simulink model "simF16_u02"  (R2023b)
settings: Solver=ode4  StartTime=0  StopTime=15  FixedStep=0.005  RelTol=1e-3  EnableMultiTasking=on
values from neighbouring files (symbols this model uses):
  control_trim = u0    [find_trim.m]    (also in trimcond.mat = [0.154059600013 -0.694715670316 -3.42749873112e-15 4.5481145; trimcond2.mat = [0.154007747083 -0.694801754663 0.00182544197392 0.000329744)
  state_trim = constraint( state )    [find_trim.m]    (also in trimcond.mat = [502 0.0505701217863 2.65111802467e-16 0 0.0505701217863 0 0; trimcond2.mat = [501.999976668 0.0505473192089 -2.30406790676e-05 0.00010278)
settings Model: Creator=keviczky  LastModifiedBy=suvo
settings DataIOCC: Decimation=50  SaveFormat=Array  SignalLoggingSaveFormat=ModelDataLogs  ReturnWorkspaceOutputs=off  SignalLoggingName=sigsOut
settings OptimizationCC: BooleanDataType=off
settings DebuggingCC: SaveWithParameterizedLinksMsg=none  UnderspecifiedInitializationDetection=Classic  MergeDetectMultiDrivingBlocksExec=none  SignalResolutionControl=TryResolveAllWithWarning  MultiTaskDSMMsg=warning  MultiTaskCondExecSysMsg=none  UnconnectedInputMsg=warning  UnconnectedOutputMsg=warning  UnconnectedLineMsg=warning
settings HardwareCC: ProdBitPerPointer=32  ProdBitPerSizeT=32  ProdBitPerPtrDiffT=32  ProdLargestAtomicFloat=None  ProdIntDivRoundTo=Undefined  ProdEndianess=Unspecified  ProdWordSize=32  ProdHWDeviceType=32-bit Generic  TargetUnknown=on
settings ModelReferenceCC: PropagateSignalLabelsOutOfModel=off
settings GRTTargetCC: CombineOutputUpdateFcns=off  GRTInterface=on
settings ConfigComp: CovMetricSettings=dw  CovSaveCumulativeToWorkspaceVar=on  CovSaveSingleToWorkspaceVar=on

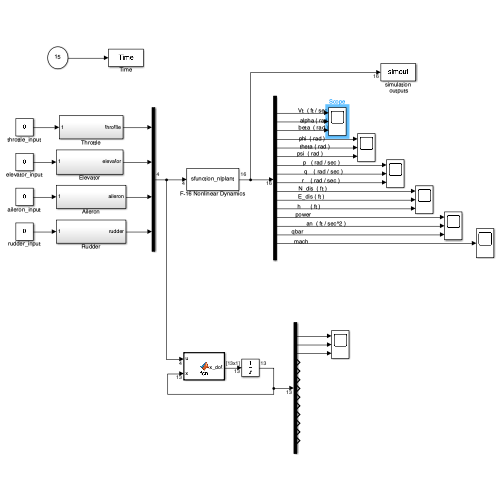
[thumbnail: Simulink's stored preview of the top-level diagram]
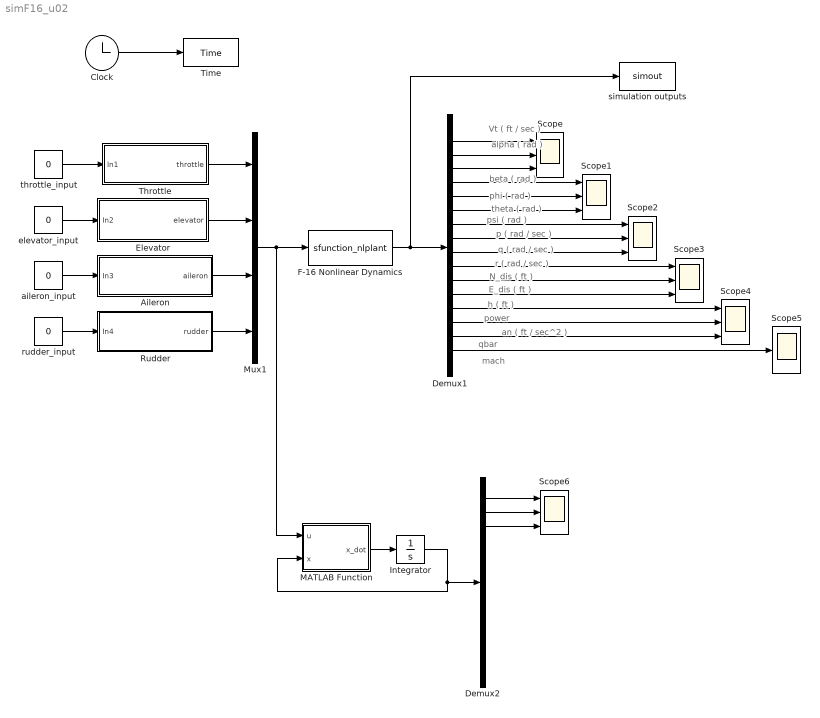
== system simF16_u02 ==
  note: Vt ( ft / sec )
  note: alpha ( rad )
  note: beta ( rad )
  note: phi ( rad )
  note: theta ( rad )
  note: psi ( rad )
  note: p ( rad / sec )
  note: q ( rad / sec )
  note: r ( rad / sec )
  note: N_dis ( ft )
  note: E_dis ( ft )
  note: h ( ft )
  note: power
  note: an ( ft / sec^2 )
  note: qbar
  note: mach
  Aileron : Subsystem
  Clock : Clock
      settings: Decimation=50
  Demux1 : Demux  Outputs=16
  Demux2 : Demux  Outputs=13
  Elevator : Subsystem
  F-16 Nonlinear Dynamics : S-Function  FunctionName=sfunction_nlplant  Parameters="state_trim,  xcg"  SFunctionDeploymentMode=off  EnableBusSupport=off
  Integrator : Integrator  InitialCondition=[state_trim]
  MATLAB Function : MATLAB Function  TreatAsAtomicUnit=on
  Mux1 : Mux
  Rudder : Subsystem
  Scope{,1..4,6} (6 alike) : Scope  NumInputPorts=3
  Scope5 : Scope
  Throttle : Subsystem
  Time : ToWorkspace  VariableName=Time  SampleTime=-1
      settings: Decimation=100
  aileron_input : Constant  Value=0
  elevator_input : Constant  Value=0
  rudder_input : Constant  Value=0
  simulation outputs : ToWorkspace  VariableName=simout  SampleTime=-1
      settings: Decimation=100
  throttle_input : Constant  Value=0
  wires:
  F-16 Nonlinear Dynamics/1 -> Demux1/1, simulation outputs/1
  Clock/1 -> Time/1
  Demux1/1 -> Scope/1
  Demux1/2 -> Scope/2
  Demux1/3 -> Scope/3
  Demux1/5 -> Scope1/2
  Demux1/6 -> Scope1/3
  Demux1/7 -> Scope2/1
  Demux1/8 -> Scope2/2
  Demux1/9 -> Scope2/3
  Demux1/10 -> Scope3/1
  Demux1/11 -> Scope3/2
  Demux1/12 -> Scope3/3
  Demux1/13 -> Scope4/1
  Demux1/14 -> Scope4/2
  Demux1/4 -> Scope1/1
  Demux1/15 -> Scope4/3
  Demux1/16 -> Scope5/1
  Throttle/1(throttle) -> Mux1/1
  Elevator/1(elevator) -> Mux1/2
  Aileron/1(aileron) -> Mux1/3
  Rudder/1(rudder) -> Mux1/4
  throttle_input/1 -> Throttle/1(In1)
  elevator_input/1 -> Elevator/1(In2)
  aileron_input/1 -> Aileron/1(In3)
  rudder_input/1 -> Rudder/1(In4)
  MATLAB Function/1(x_dot) -> Integrator/1
  Integrator/1 -> MATLAB Function/2(x), Demux2/1
  Mux1/1 -> MATLAB Function/1(u), F-16 Nonlinear Dynamics/1
  Demux2/1 -> Scope6/1
  Demux2/2 -> Scope6/2
  Demux2/3 -> Scope6/3

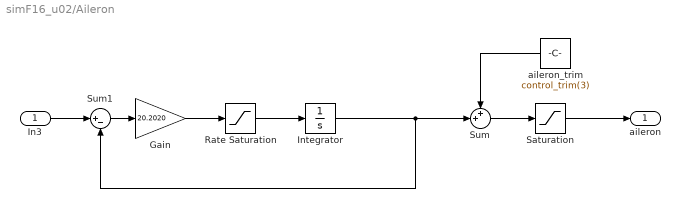
== system simF16_u02/Aileron ==
  In3 : Inport
  Gain : Gain  Gain=20.2020  SaturateOnIntegerOverflow=on  OutDataTypeStr=Inherit: Same as input  ParamDataTypeStr=Inherit: Same as input
  Integrator : Integrator  UpperSaturationLimit=21.5  LowerSaturationLimit=-21.5
  Rate Saturation : Saturate  UpperLimit=80  LowerLimit=-80
  Saturation : Saturate  UpperLimit=21.5  LowerLimit=-21.5
  Sum : Sum  Inputs=++|  InputSameDT=on  SaturateOnIntegerOverflow=on  OutDataTypeStr=Inherit: Same as first input
  Sum1 : Sum  Inputs=|+-  InputSameDT=on  SaturateOnIntegerOverflow=on  OutDataTypeStr=Inherit: Same as first input
  aileron_trim : Constant  Value=control_trim(3)
  aileron : Outport
  wires:
  In3/1 -> Sum1/1
  Sum1/1 -> Gain/1
  Gain/1 -> Rate Saturation/1
  Rate Saturation/1 -> Integrator/1
  Integrator/1 -> Sum1/2, Sum/2
  Sum/1 -> Saturation/1
  aileron_trim/1 -> Sum/1
  Saturation/1 -> aileron/1

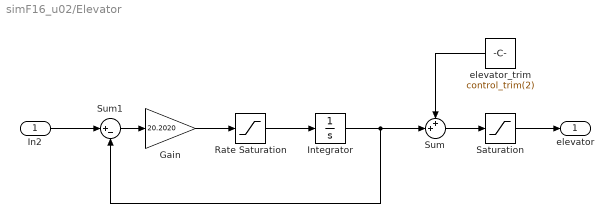
== system simF16_u02/Elevator ==
  In2 : Inport
  Gain : Gain  Gain=20.2020  SaturateOnIntegerOverflow=on  OutDataTypeStr=Inherit: Same as input  ParamDataTypeStr=Inherit: Same as input
  Integrator : Integrator  UpperSaturationLimit=25  LowerSaturationLimit=-25
  Rate Saturation : Saturate  UpperLimit=60  LowerLimit=-60
  Saturation : Saturate  UpperLimit=25  LowerLimit=-25
  Sum : Sum  Inputs=++|  InputSameDT=on  SaturateOnIntegerOverflow=on  OutDataTypeStr=Inherit: Same as first input
  Sum1 : Sum  Inputs=|+-  InputSameDT=on  SaturateOnIntegerOverflow=on  OutDataTypeStr=Inherit: Same as first input
  elevator_trim : Constant  Value=control_trim(2)
  elevator : Outport
  wires:
  In2/1 -> Sum1/1
  Sum1/1 -> Gain/1
  Gain/1 -> Rate Saturation/1
  Rate Saturation/1 -> Integrator/1
  Integrator/1 -> Sum1/2, Sum/2
  Sum/1 -> Saturation/1
  elevator_trim/1 -> Sum/1
  Saturation/1 -> elevator/1

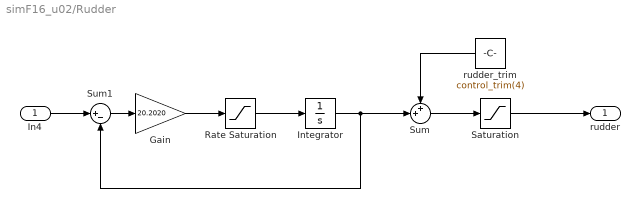
== system simF16_u02/Rudder ==
  In4 : Inport
  Gain : Gain  Gain=20.2020  SaturateOnIntegerOverflow=on  OutDataTypeStr=Inherit: Same as input  ParamDataTypeStr=Inherit: Same as input
  Integrator : Integrator  UpperSaturationLimit=30  LowerSaturationLimit=-30
  Rate Saturation : Saturate  UpperLimit=120  LowerLimit=-120
  Saturation : Saturate  UpperLimit=30  LowerLimit=-30
  Sum : Sum  Inputs=++|  InputSameDT=on  SaturateOnIntegerOverflow=on  OutDataTypeStr=Inherit: Same as first input
  Sum1 : Sum  Inputs=|+-  InputSameDT=on  SaturateOnIntegerOverflow=on  OutDataTypeStr=Inherit: Same as first input
  rudder_trim : Constant  Value=control_trim(4)
  rudder : Outport
  wires:
  In4/1 -> Sum1/1
  Sum1/1 -> Gain/1
  Gain/1 -> Rate Saturation/1
  Rate Saturation/1 -> Integrator/1
  Integrator/1 -> Sum1/2, Sum/2
  Saturation/1 -> rudder/1
  Sum/1 -> Saturation/1
  rudder_trim/1 -> Sum/1

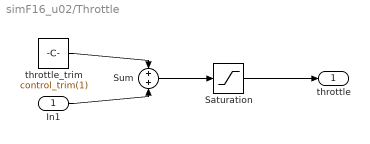
== system simF16_u02/Throttle ==
  In1 : Inport
  Saturation : Saturate  UpperLimit=1  LowerLimit=0
  Sum : Sum  InputSameDT=on  SaturateOnIntegerOverflow=on  OutDataTypeStr=Inherit: Same as first input
  throttle_trim : Constant  Value=control_trim(1)
  throttle : Outport
  wires:
  throttle_trim/1 -> Sum/1
  In1/1 -> Sum/2
  Sum/1 -> Saturation/1
  Saturation/1 -> throttle/1

== matlab function simF16_u02/MATLAB Function ==
  data: u input; x input; x_dot output
function x_dot = fcn(u,x)
%% ---- constant variable ----------------
s = 300;
b = 30;
cbar = 11.32;
rm = 1.57e-3; % 1 / mass
xcgr = 0.35;
he = 160.0;

x_dot = zeros(13,1);
xcg = 0.35;
control = u;

%% ---- Inertia constants ----------------
c1 = -0.770;
c2 = 0.02755;
c3 = 1.055e-4;
c4 = 1.642e-6;
c5 = 0.9604;
c6 = 1.759e-2;
c7 = 1.792e-5;
c8 = -0.7336;
c9 = 1.587e-5;

rtod = 180 / pi; %% radians to degrees
g = 32.174;

%% ---- Assign state variables ---------------
vt = x(1);
alpha = x(2) * rtod; %% x(2) in radians, alpha in degrees.
beta = x(3) * rtod;  %% x(3) in radians, beta in degrees.
phi = x(4);
theta = x(5);
psi = x(6);
p = x(7);
q = x(8);
r = x(9);
alt = x(12);
pow = x(13); % power

%% ---- Assign state & control variables ---------------
thtl = control(1);
el   = control(2);
ail  = control(3);
rdr  = control(4);

%% ---- Air Data computer and engine model ------------
[tfac, t, rho, amach, qbar, ps ] = adc ( vt, alt ); 
cpow = tgear (thtl);
x_dot (13) = pdot ( pow, cpow );  %% x_dot(13) = power derivative
t = thrust ( pow, alt, amach );

%% ---- Look-up tables and component biuldup ------------
cxt = cx ( alpha, el );
cyt = cy ( beta, ail, rdr );
czt = cz ( alpha, beta, el );
dail = ail / 20.0;
drdr = rdr / 30.0;
dlda_value = dlda( alpha, beta );
dldr_value = dldr( alpha, beta );
clt = cl( alpha, beta ) + dlda_value * dail + dldr_value * drdr;
cmt = cm( alpha, el );
dnda_value = dnda( alpha, beta );
dndr_value = dndr( alpha, beta );
cnt = cn( alpha, beta ) + dnda_value * dail + dndr_value * drdr;

%% ---- Add damping derivatives ------------
tvt = 0.5 / vt;
b2v = b * tvt;
cq = cbar * q * tvt;
d = damping( alpha );
cxt = cxt + cq * d(1);
cyt = cyt + b2v * ( d(2) * r + d(3) * p );
czt = czt + cq * d(4);
clt = clt + b2v * ( d(5) * r + d(6) * p );
cmt = cmt + cq * d(7) + czt * ( xcgr - xcg );
cnt = cnt + b2v * ( d(8)* r + d(9) * p ) - cyt * ( xcgr - xcg ) * cbar / b;

%% ---- Get ready for state equations ------------
cbta = cos( x(3) );
u = vt * cos( x(2) ) * cbta;
v = vt * sin( x(3) );
w = vt * sin( x(2) ) * cbta;
sth = sin( theta );
cth = cos( theta );
sph = sin( phi );
cph = cos( phi );
spsi = sin( psi );
cpsi = cos( psi );
qs = qbar * s;
qsb = qs * b;
rmqs = rm *qs;
gcth = g * cth;
qsph = q * sph;
ay = rmqs * cyt;
az = rmqs * czt;

%% ---- Force equations ------------
udot = r * v - q * w - g * sth + rm * ( qs * cxt + t );
vdot = p * w - r * u + gcth * sph + ay;
wdot = q * u - p * v + gcth * cph + az;
dum = ( u * u + w * w );
x_dot(1) = ( u * udot + v * vdot + w * wdot ) / vt;
x_dot(2) = (u * wdot - w * udot ) / dum;
x_dot(3) = (vt * vdot - v * x_dot(1) ) * cbta / dum;

%% ---- Kinematics ------------
x_dot(4) = p + ( sth / cth ) * (qsph + r * cph );
x_dot(5) = q * cph - r * sph;
x_dot(6) = ( qsph + r * cph ) / cth;

%% ---- Moments ------------
x_dot(7) = ( c2 * p + c1 * r + c4 * he ) * q + qsb * ( c3 * clt + c4 * cnt );
x_dot(8) = ( c5 * p -c7 * he )* r + c6 * ( r^2 - p^2 ) + qs * cbar * c7 * cmt;
x_dot(9) = ( c8 * p - c2 * r + c9 * he ) * q + qsb * ( c4 * clt + c9 * cnt );

%% ---- Mavigation ------------
t1 = sph * cpsi;
t2 = cph * sth;
t3 = sph * spsi;
s1 = cth * cpsi;
s2 = cth * spsi;
s3 = t1 * sth - cph * spsi;
s4 = t3 * sth + cph * cpsi;
s5 = sph * cth;
s6 = t2 * cpsi + t3;
s7 = t2 * spsi - t1;
s8 = cph * cth;

x_dot(10) = u * s1 + v * s3 + w * s6;  %% north speed
x_dot(11) = u * s2 + v * s4 + w * s7;  %% east speed
x_dot(12) = u * sth - v * s5 - w * s8; %% vertical speed

%x_dot = x_dot'; % transfer the vector to a column vector
